simulink model "simulink_1"  (R2021a)
settings: Solver=VariableStepAuto  StartTime=0.0  StopTime=10.0  RelTol=1e-3
settings Model: Creator=Pavilion  LastModifiedBy=Pavilion

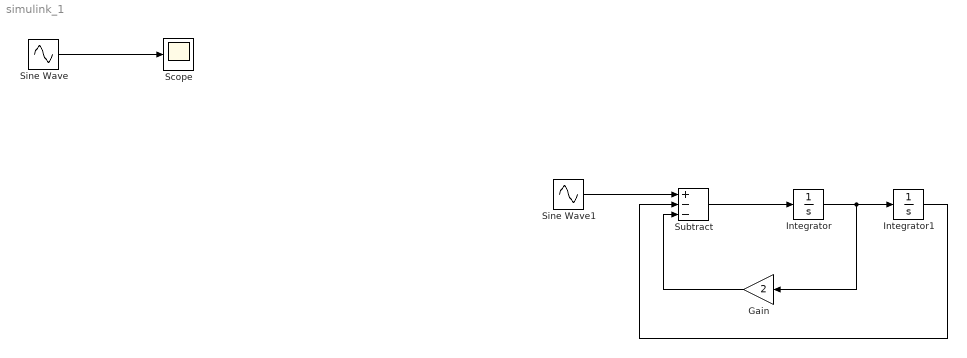
== system simulink_1 ==
  Gain : Gain  Gain=2
  Integrator : Integrator
  Integrator1 : Integrator
  Scope : Scope
  Sine Wave : Sin  Frequency=2  SampleTime=0
  Sine Wave1 : Sin  Frequency=2  SampleTime=0
  Subtract : Sum  Inputs=+--
  wires:
  Sine Wave/1 -> Scope/1
  Subtract/1 -> Integrator/1
  Integrator/1 -> Gain/1, Integrator1/1
  Sine Wave1/1 -> Subtract/1
  Gain/1 -> Subtract/3
  Integrator1/1 -> Subtract/2
